simulink model "c_to_ri_blk"  (R2019a)
settings: Solver=VariableStepAuto  StartTime=0.0  StopTime=10.0  RelTol=1e-3
libraries: xbsIndex_r4 x1
settings Model: Creator=mybur  LastModifiedBy=mybur

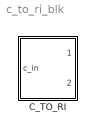
== system c_to_ri_blk ==
  C_TO_RI : Subsystem  mask{bit_width=4, bin_pt=0, is_async=off}
      mask prompts: bit_width "Bit Width"; bin_pt "Binary Point"; is_async "Asynchronous"

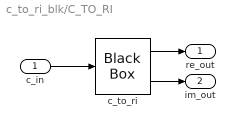
== system c_to_ri_blk/C_TO_RI ==
  c_in : Inport
  c_to_ri : xbsIndex_r4/Black Box  init_code=c_to_ri_config  sim_method=ISE Simulator  verbose=off  block_type=blackbox2
  re_out : Outport
  im_out : Outport  Port=2
  wires:
  c_in/1 -> c_to_ri/1
  c_to_ri/1 -> re_out/1
  c_to_ri/2 -> im_out/1
